simulink model "model_lqr_TODO_2017b"  (R2017b)
settings: Solver=VariableStepAuto  StartTime=0.0  StopTime=10.0  RelTol=1e-3
values from neighbouring files (symbols this model uses):
  f = [0 0 1 0 ... (first row only)    [Main.m]
  g = [0 0 ... (first row only)    [Main.m]
undefined symbols (not defined in the file or in its folder): K_lqr
settings Model: Creator=Victus  LastModifiedBy=Victus
settings DataIOCC: ReturnWorkspaceOutputs=on
settings DebuggingCC: UnconnectedInputMsg=none  UnconnectedOutputMsg=none  UnconnectedLineMsg=none
settings ModelReferenceCC: EnableRefExpFcnMdlSchedulingChecks=off
settings SFSimCC: SimUseLocalCustomCode=on
settings RTWCC: Description=Generic Real-Time Target  RTWUseLocalCustomCode=on

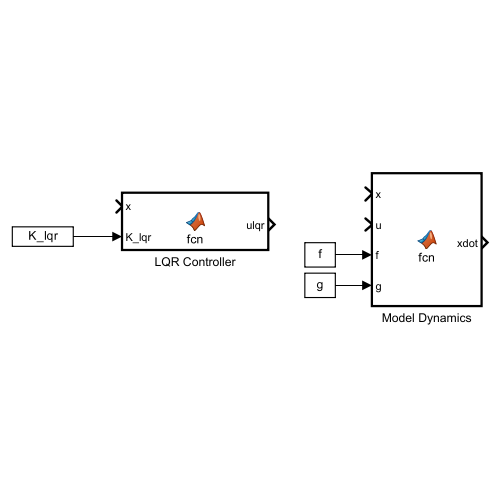
[thumbnail: Simulink's stored preview of the top-level diagram]
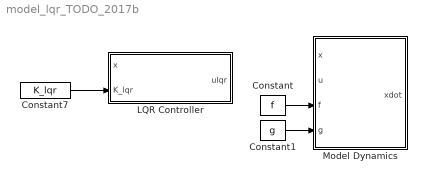
== system model_lqr_TODO_2017b ==
  Constant : Constant  Value=f
  Constant1 : Constant  Value=g
  Constant7 : Constant  Value=K_lqr
  LQR Controller : MATLAB Function  TreatAsAtomicUnit=on
  Model Dynamics : MATLAB Function  TreatAsAtomicUnit=on
  wires:
  Constant7/1 -> LQR Controller/2(K_lqr)
  Constant1/1 -> Model Dynamics/4(g)
  Constant/1 -> Model Dynamics/3(f)

== matlab function model_lqr_TODO_2017b/Model Dynamics ==
  data: x input; u input; xdot output; f input; g input
function xdot = fcn(x,u,f,g)
    xdot = f*x + g*u;
end

== matlab function model_lqr_TODO_2017b/LQR Controller ==
  data: x input; ulqr output; K_lqr input
function ulqr = fcn(x,K_lqr)
    ulqr = -K_lqr*x;
end
